simulink model "ARDroneWPTrackingSimulationRedBull"  (R2018b)
settings: Solver=ode1  StartTime=0.0  StopTime=150  FixedStep=t_samp  RelTol=1e-3  EnableMultiTasking=on
undefined symbols (not defined in the file): Gxd_A_obs, Gxd_B_obs, Gxd_C_obs, Gyawd_A_obs, Gyawd_B_obs, Gyawd_C_obs, Gyd_A_obs, Gyd_B_obs, Gyd_C_obs, Gzd_A_obs, Gzd_B_obs, Gzd_C_obs, K0_X, K0_Y, K0_yaw, K0_Z, K_X, K_Y, K_yaw, K_Z, KGe_X, KGe_Y, KGe_yaw, KGe_Z, ssH, ssPitch, ssPitch2U, ssRoll, ssRoll2V, ssYaw, t_samp, waypoint
libraries: simulink x3
CloseFcn:
  | rtwprivate ssgencode ModelCloseRequest Good_NL_model
settings Model: ExtModeTrigDuration=100000  Creator=Paul  LastModifiedBy=Henrique
settings DataIOCC: LimitDataPoints=on  SaveFormat=Array  TimeSaveName=time
settings OptimizationCC: ExpressionDepthLimit=2147483647  InitFltsAndDblsToZero=on
settings DebuggingCC: UnderspecifiedInitializationDetection=Classic  MergeDetectMultiDrivingBlocksExec=none  SolverPrmCheckMsg=warning  FcnCallInpInsideContextMsg=warning  StateNameClashWarn=warning  SFUnexpectedBacktrackingDiag=warning  SFNoUnconditionalDefaultTransitionDiag=warning  SFExecutionAtInitializationDiag=none
settings ModelReferenceCC: PropagateSignalLabelsOutOfModel=off
settings SFSimCC: SimUseLocalCustomCode=off
settings RTWCC: SystemTargetFile=sldrt.tlc  TemplateMakefile=sldrt.tmf  Description=Simulink Desktop Real-Time  RTWUseLocalCustomCode=off  RTWCompilerOptimization=on
settings CodeAppCC: MaxIdLength=95  StateflowObjectComments=on
settings SimulinkDesktopRealTimeCC: TargetPreCompLibLocation=D:\Programas\MATLAB 2018b\toolbox\sldrt\lib\win64  TargetLangStandard=C89/C90 (ANSI)  SupportVariableSizeSignals=off  PreserveStateflowLocalDataDimensions=off
settings ConfigComp: CovMetricSettings=dw  CovHtmlReporting=on  CovSaveCumulativeToWorkspaceVar=on  CovSaveSingleToWorkspaceVar=on  CovExternalEMLEnable=off

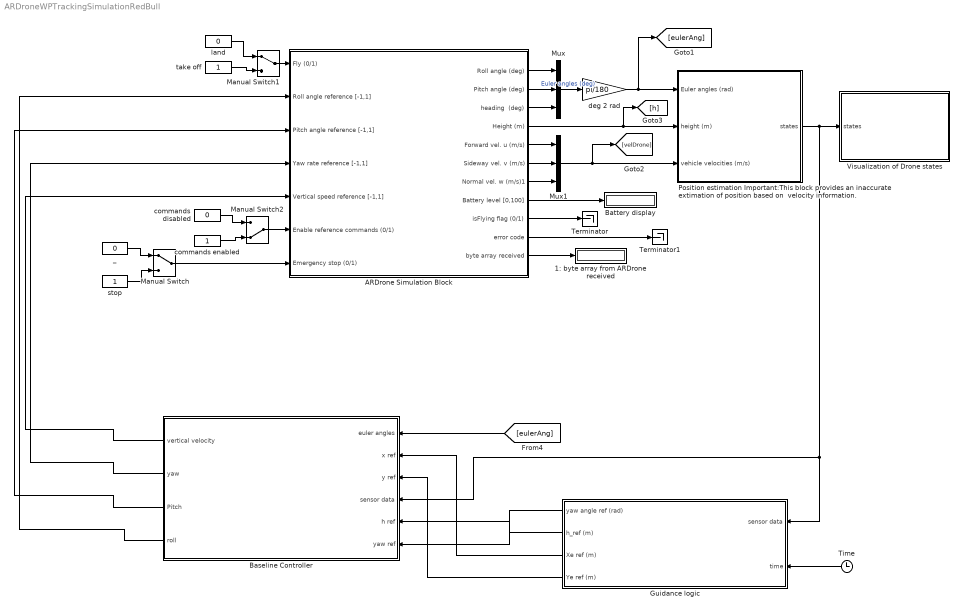
== system ARDroneWPTrackingSimulationRedBull ==
  "1: byte array from ARDrone received " : Display
  ARDrone Simulation Block : Subsystem  AncestorBlock=ARBlocks/ARDrone Simulation Block
  Baseline Controller : Subsystem  AncestorBlock=ARBlocks/Baseline Controller
  Battery display : Display
  Guidance logic : Subsystem  AncestorBlock=ARBlocks/Guidance logic
  Manual Switch : ManualSwitch
  Manual Switch1 : ManualSwitch
  Manual Switch2 : ManualSwitch  CurrentSetting=0
  Mux : Mux  Inputs=3
  Mux1 : Mux  Inputs=3
  "Position estimation Important:This block provides an inaccurate extimation of position based on  velocity information. " : Subsystem  AncestorBlock=|
      | ARBlocks/Position estimation
      | Important:This block provides an 
      | inaccurate extimation of position 
      | based on  velocity information.
  Terminator : Terminator
  Terminator1 : Terminator
  Time : Clock
  Visualization of Drone states : Subsystem
  _ : Constant  Value=0
  commands disabled : Constant  Value=0
  commands enabled : Constant
  deg 2 rad : Gain  Gain=pi/180
  land : Constant  Value=0
  stop : Constant
  take off : Constant
  wires:
  _/1 -> Manual Switch/1
  stop/1 -> Manual Switch/2
  land/1 -> Manual Switch1/1
  take off/1 -> Manual Switch1/2
  commands disabled/1 -> Manual Switch2/1
  commands enabled/1 -> Manual Switch2/2
  Manual Switch1/1 -> ARDrone Simulation Block/1(Fly (0/1))
  Manual Switch2/1 -> ARDrone Simulation Block/6(Enable reference commands (0/1))
  Manual Switch/1 -> ARDrone Simulation Block/7(Emergency stop (0/1))
  ARDrone Simulation Block/1(Roll angle (deg)) -> Mux/1
  ARDrone Simulation Block/2(Pitch angle (deg)) -> Mux/2
  ARDrone Simulation Block/5(Forward vel. u (m/s)) -> Mux1/1
  ARDrone Simulation Block/6(Sideway vel. v (m/s)) -> Mux1/2
  ARDrone Simulation Block/7(Normal vel. w (m/s)1) -> Mux1/3
  Mux/1 -> deg 2 rad/1  "Euler angles (deg)"
  ARDrone Simulation Block/8(Battery level [0,100]) -> Battery display/1
  deg 2 rad/1 -> "Position estimation Important:This block provides an inaccurate extimation of position based on  velocity information. "/1(Euler angles (rad)), [eulerAng]
  ARDrone Simulation Block/4(Height (m)) -> [h], "Position estimation Important:This block provides an inaccurate extimation of position based on  velocity information. "/2(height (m))
  ARDrone Simulation Block/3(heading  (deg)) -> Mux/3
  ARDrone Simulation Block/9(isFlying flag (0/1)) -> Terminator/1
  ARDrone Simulation Block/10(error code) -> Terminator1/1
  ARDrone Simulation Block/11(byte array received) -> "1: byte array from ARDrone received "/1
  "Position estimation Important:This block provides an inaccurate extimation of position based on  velocity information. "/1(states) -> Baseline Controller/4(sensor data), Guidance logic/1(sensor data), Visualization of Drone states/1(states)
  Mux1/1 -> [velDrone], "Position estimation Important:This block provides an inaccurate extimation of position based on  velocity information. "/3(vehicle velocities (m/s))
  [eulerAng] -> Baseline Controller/1(euler angles)
  Time/1 -> Guidance logic/2(time)
  Guidance logic/3(Xe ref (m)) -> Baseline Controller/2(x ref)
  Guidance logic/4(Ye ref (m)) -> Baseline Controller/3(y ref)
  Baseline Controller/1("vertical velocity ") -> ARDrone Simulation Block/5(Vertical speed reference [-1,1])
  Baseline Controller/2("yaw ") -> ARDrone Simulation Block/4(Yaw rate reference [-1,1])
  Baseline Controller/3("Pitch ") -> ARDrone Simulation Block/3(Pitch angle reference [-1,1])
  Baseline Controller/4("roll ") -> ARDrone Simulation Block/2(Roll angle reference [-1,1])
  Guidance logic/2(h_ref (m)) -> Baseline Controller/5(h ref)
  Guidance logic/1(yaw angle ref (rad)) -> Baseline Controller/6(yaw ref)

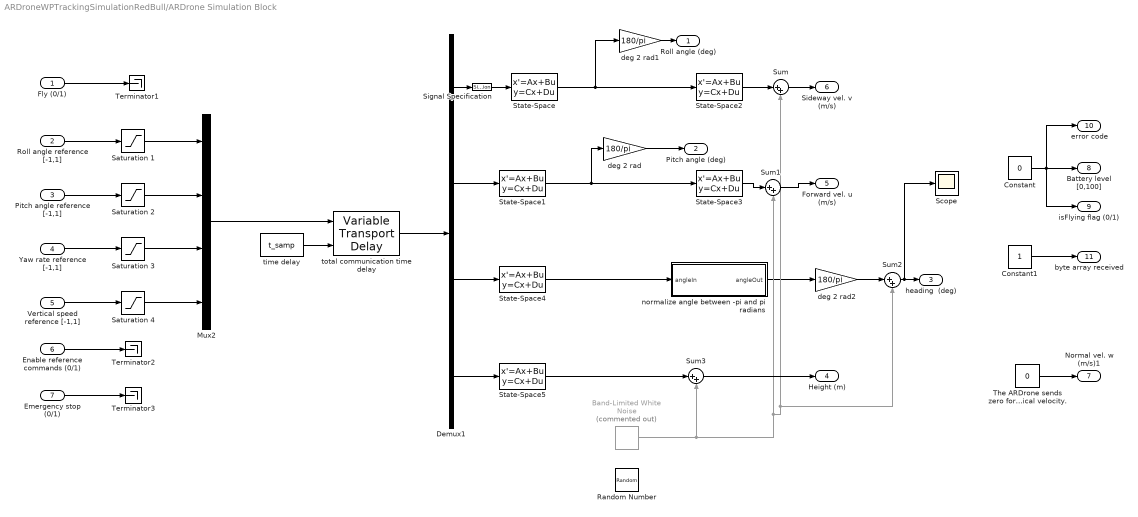
== system ARDroneWPTrackingSimulationRedBull/ARDrone Simulation Block ==
  Fly (0/1) : Inport
  Roll angle reference [-1,1] : Inport  Port=2
  Pitch angle reference [-1,1] : Inport  Port=3
  Yaw rate reference [-1,1] : Inport  Port=4
  Vertical speed reference [-1,1] : Inport  Port=5
  Enable reference commands (0/1) : Inport  Port=6
  Emergency stop (0/1) : Inport  Port=7
  Band-Limited White Noise : simulink/Sources/Band-Limited White Noise  Commented=on  Cov=[0.1]  Ts=0.065  seed=[23341]
  Constant : Constant  Value=0
  Constant1 : Constant
  Demux1 : Demux
  Mux2 : Mux
  Random Number : RandomNumber  SampleTime=0.065
  Saturation {1..4} (4 alike) : Saturate  UpperLimit=1  LowerLimit=-1
  Scope : Scope
  Signal Specification : SignalSpecification  Dimensions=1
  State-Space : StateSpace  A=ssRoll.a  B=ssRoll.b  C=ssRoll.c  D=ssRoll.d  InitialCondition=0
  State-Space1 : StateSpace  A=ssPitch.a  B=ssPitch.b  C=ssPitch.c  D=ssPitch.d  InitialCondition=0
  State-Space2 : StateSpace  A=ssRoll2V.a  B=ssRoll2V.b  C=ssRoll2V.c  D=ssRoll2V.d  InitialCondition=0
  State-Space3 : StateSpace  A=ssPitch2U.a  B=ssPitch2U.b  C=ssPitch2U.c  D=ssPitch2U.d  InitialCondition=0
  State-Space4 : StateSpace  A=ssYaw.a  B=ssYaw.b  C=ssYaw.c  D=ssYaw.d  InitialCondition=0
  State-Space5 : StateSpace  A=ssH.a  B=ssH.b  C=ssH.c  D=ssH.d  InitialCondition=0
  Sum{,1..3} (4 alike) : Sum  Inputs=|++
  Terminator1 : Terminator
  Terminator2 : Terminator
  Terminator3 : Terminator
  "The ARDrone sends zero for the vertical velocity. " : Constant  Value=0
  deg 2 rad : Gain  Gain=180/pi
  deg 2 rad1 : Gain  Gain=180/pi
  deg 2 rad2 : Gain  Gain=180/pi
  normalize angle between -pi and pi radians : MATLAB Function  TreatAsAtomicUnit=on
  time delay : Constant  Value=t_samp
  total communication time delay : VariableTransportDelay  MaximumDelay=10  InitialOutput=[0 0 0 0]  MaximumPoints=4096
  Roll angle (deg) : Outport
  Pitch angle (deg) : Outport  Port=2
  heading  (deg) : Outport  Port=3
  Height (m) : Outport  Port=4
  Forward vel. u (m/s) : Outport  Port=5
  Sideway vel. v (m/s) : Outport  Port=6
  Normal vel. w (m/s)1 : Outport  Port=7
  Battery level [0,100] : Outport  Port=8
  isFlying flag (0/1) : Outport  Port=9
  error code : Outport  Port=10
  byte array received : Outport  Port=11
  wires:
  "The ARDrone sends zero for the vertical velocity. "/1 -> Normal vel. w (m/s)1/1
  Constant1/1 -> byte array received/1
  deg 2 rad1/1 -> Roll angle (deg)/1
  deg 2 rad/1 -> Pitch angle (deg)/1
  Constant/1 -> Battery level [0,100]/1, error code/1, isFlying flag (0/1)/1
  normalize angle between -pi and pi radians/1(angleOut) -> deg 2 rad2/1
  Emergency stop (0/1)/1 -> Terminator3/1
  Enable reference commands (0/1)/1 -> Terminator2/1
  Fly (0/1)/1 -> Terminator1/1
  State-Space4/1 -> normalize angle between -pi and pi radians/1(angleIn)
  Demux1/3 -> State-Space4/1
  Demux1/2 -> State-Space1/1
  Saturation 4/1 -> Mux2/4
  Saturation 3/1 -> Mux2/3
  Saturation 2/1 -> Mux2/2
  Saturation 1/1 -> Mux2/1
  total communication time delay/1 -> Demux1/1
  Mux2/1 -> total communication time delay/1
  time delay/1 -> total communication time delay/2
  State-Space1/1 -> State-Space3/1, deg 2 rad/1
  State-Space/1 -> State-Space2/1, deg 2 rad1/1
  Demux1/4 -> State-Space5/1
  Vertical speed reference [-1,1]/1 -> Saturation 4/1
  Yaw rate reference [-1,1]/1 -> Saturation 3/1
  Pitch angle reference [-1,1]/1 -> Saturation 2/1
  Roll angle reference [-1,1]/1 -> Saturation 1/1
  Demux1/1 -> Signal Specification/1
  Signal Specification/1 -> State-Space/1
  State-Space2/1 -> Sum/1
  Sum/1 -> Sideway vel. v (m/s)/1
  Band-Limited White Noise/1 -> Sum3/2, Sum1/2, Sum2/2, Sum/2
  State-Space3/1 -> Sum1/1
  Sum1/1 -> Forward vel. u (m/s)/1
  Sum2/1 -> Scope/1, heading  (deg)/1
  deg 2 rad2/1 -> Sum2/1
  State-Space5/1 -> Sum3/1
  Sum3/1 -> Height (m)/1

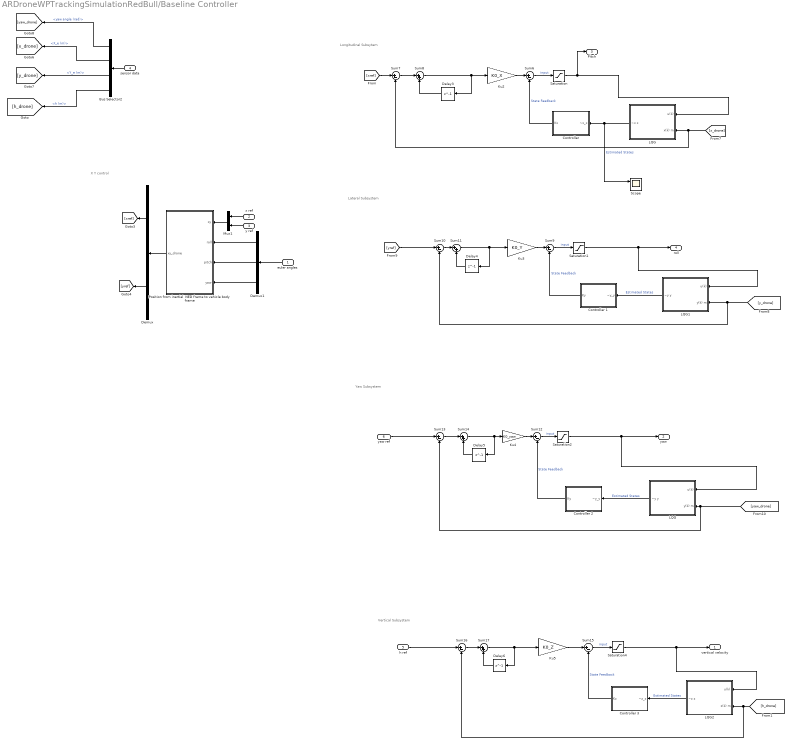
== system ARDroneWPTrackingSimulationRedBull/Baseline Controller ==
  note: Vertical Subsystem
  note: Yaw Subsystem
  note: Lateral Subsystem
  note: Longitudinal Subsytem
  note: X Y control
  euler angles : Inport
  x ref : Inport  Port=2
  y ref : Inport  Port=3
  sensor data : Inport  Port=4
  h ref : Inport  Port=5
  yaw ref : Inport  Port=6
  Bus Selector2 : BusSelector  OutputSignals=yaw angle (rad),X_e (m),Y_e (m),h (m)
  "Controller " : Subsystem
  Controller 1 : Subsystem
  Controller 2 : Subsystem
  Controller 3 : Subsystem
  Delay{3..6} (4 alike) : Delay  DelayLength=1  InitialCondition=0
  Demux : Demux  Outputs=2
  Demux1 : Demux  Outputs=3
  Ku2 : Gain  Gain=K0_X
  Ku3 : Gain  Gain=K0_Y
  Ku4 : Gain  Gain=K0_yaw
  Ku5 : Gain  Gain=K0_Z
  LQG : Subsystem
  "LQG " : Subsystem
  LQG1 : Subsystem
  LQG2 : Subsystem
  Mux1 : Mux  Inputs=2
  Position from inertial  NED frame to vehicle body frame : MATLAB Function  TreatAsAtomicUnit=on
  Saturation : Saturate  UpperLimit=2  LowerLimit=-1.2
  Saturation1 : Saturate  UpperLimit=1.2  LowerLimit=-1.2
  Saturation2 : Saturate  UpperLimit=1.2  LowerLimit=-1.2
  Saturation4 : Saturate  UpperLimit=1.2  LowerLimit=-1.2
  Scope : Scope  NumInputPorts=2
  Sum{6..7,9..10,12..13,15..16} (8 alike) : Sum  Inputs=|+-
  Sum{8,11,14,17} (4 alike) : Sum  Inputs=|++
  "vertical velocity " : Outport
  "yaw " : Outport  Port=2
  "Pitch " : Outport  Port=3
  "roll " : Outport  Port=4
  wires:
  Mux1/1 -> Position from inertial  NED frame to vehicle body frame/1(xy)
  x ref/1 -> Mux1/1
  y ref/1 -> Mux1/2
  Position from inertial  NED frame to vehicle body frame/1(xy_drone) -> Demux/1
  Demux1/1 -> Position from inertial  NED frame to vehicle body frame/2(roll)
  Demux1/2 -> Position from inertial  NED frame to vehicle body frame/3(pitch)
  Demux1/3 -> Position from inertial  NED frame to vehicle body frame/4(yaw)
  euler angles/1 -> Demux1/1
  Bus Selector2/1 -> [yaw_drone]  "<yaw angle (rad)>"
  Bus Selector2/3 -> [y_drone]  "<Y_e (m)>"
  sensor data/1 -> Bus Selector2/1
  Bus Selector2/4 -> [h_drone]  "<h (m)>"
  Bus Selector2/2 -> [x_drone]  "<X_e (m)>"
  Delay3/1 -> Sum8/2
  Ku2/1 -> Sum6/1
  LQG/1("~x x ") -> Scope/1, "Controller "/1(~x_x)  "Estimated States"
  "Controller "/1(Kx) -> Sum6/2  "State Feedback"
  Sum8/1 -> Ku2/1, Delay3/1
  [xref] -> Sum7/1
  Saturation/1 -> "Pitch "/1, LQG/1(u(k))
  [x_drone] -> Sum7/2, LQG/2(x(k) m)
  Sum7/1 -> Sum8/1
  Sum6/1 -> Saturation/1  "input"
  Demux/1 -> [xref]
  Ku3/1 -> Sum9/1
  Controller 1/1(Ky) -> Sum9/2  "State Feedback"
  Sum11/1 -> Delay4/1, Ku3/1
  [yref] -> Sum10/1
  Sum10/1 -> Sum11/1
  Delay4/1 -> Sum11/2
  LQG1/1("~y y ") -> Controller 1/1(~y_y)  "Estimated States"
  [y_drone] -> Sum10/2, LQG1/2(y(k) m)
  Saturation1/1 -> "roll "/1, LQG1/1(u(k))
  Sum9/1 -> Saturation1/1  "input"
  Delay5/1 -> Sum14/2
  Saturation2/1 -> "yaw "/1, "LQG "/1(u(k))
  Sum14/1 -> Delay5/1, Ku4/1
  "LQG "/1("~y y ") -> Controller 2/1(~y_y)  "Estimated States"
  Sum12/1 -> Saturation2/1  "input"
  [yaw_drone] -> Sum13/2, "LQG "/2(y(k) m)
  Ku4/1 -> Sum12/1
  Sum13/1 -> Sum14/1
  Controller 2/1(Ky) -> Sum12/2  "State Feedback"
  yaw ref/1 -> Sum13/1
  Sum17/1 -> Ku5/1, Delay6/1
  Sum16/1 -> Sum17/1
  Controller 3/1(Kz) -> Sum15/2  "State Feedback"
  Sum15/1 -> Saturation4/1  "input"
  Saturation4/1 -> "vertical velocity "/1, LQG2/1(u(k))
  LQG2/1("~z z ") -> Controller 3/1(~z_z)  "Estimated States"
  Ku5/1 -> Sum15/1
  h ref/1 -> Sum16/1
  Delay6/1 -> Sum17/2
  [h_drone] -> Sum16/2, LQG2/2(z(k) m)
  Demux/2 -> [yref]

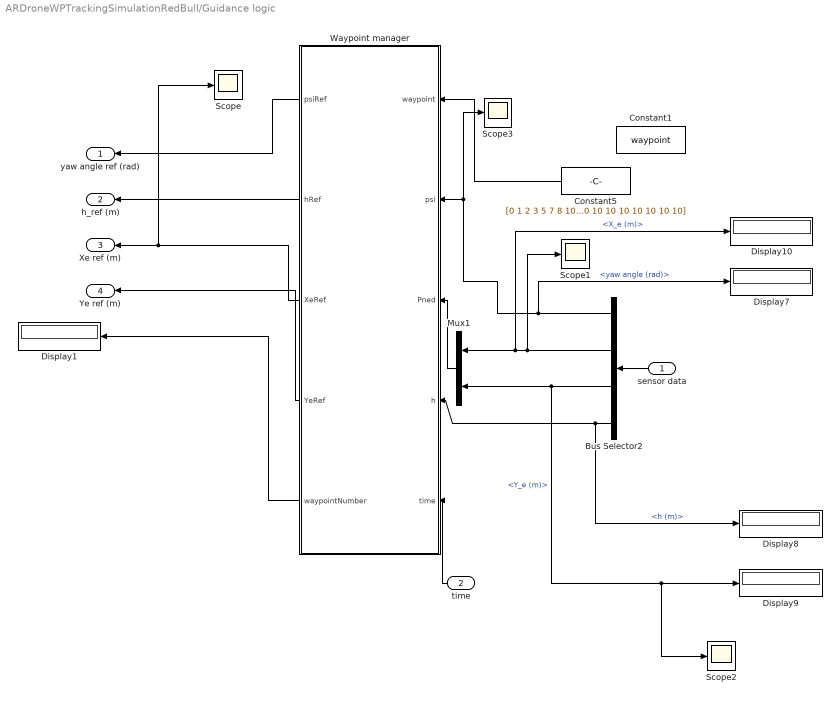
== system ARDroneWPTrackingSimulationRedBull/Guidance logic ==
  sensor data : Inport
  time : Inport  Port=2
  Bus Selector2 : BusSelector  OutputSignals=yaw angle (rad),X_e (m),Y_e (m),h (m)
  Constant1 : Constant  Value=waypoint  VectorParams1D=off
  Constant5 : Constant  Value="[0 1 2 3 5 7 8 10 11 12 13; 0 2 2 5 5 -1 -1 -2 -2 1 1; 1 2 5 2 2 1 2 3 1 1 1; 0 -0.1 0 0 0 0 0 0 0 0 0;  10 10 10 10 10 10 10 10 10 10 10]"  VectorParams1D=off
  Display{1,7..10} (5 alike) : Display
  Mux1 : Mux  Inputs=2
  Scope{,1..3} (4 alike) : Scope
  "Waypoint manager " : MATLAB Function  TreatAsAtomicUnit=on
  yaw angle ref (rad) : Outport
  h_ref (m) : Outport  Port=2
  Xe ref (m) : Outport  Port=3
  Ye ref (m) : Outport  Port=4
  wires:
  "Waypoint manager "/3(XeRef) -> Scope/1, Xe ref (m)/1
  "Waypoint manager "/5(waypointNumber) -> Display1/1
  Bus Selector2/1 -> Display7/1, Scope3/1, "Waypoint manager "/2(psi)  "<yaw angle (rad)>"
  "Waypoint manager "/1(psiRef) -> yaw angle ref (rad)/1
  Bus Selector2/2 -> Scope1/1, Mux1/1, Display10/1  "<X_e (m)>"
  Mux1/1 -> "Waypoint manager "/3(Pned)
  "Waypoint manager "/4(YeRef) -> Ye ref (m)/1
  Bus Selector2/3 -> Scope2/1, Display9/1, Mux1/2  "<Y_e (m)>"
  time/1 -> "Waypoint manager "/5(time)
  Bus Selector2/4 -> Display8/1, "Waypoint manager "/4(h)  "<h (m)>"
  Constant5/1 -> "Waypoint manager "/1(waypoint)
  "Waypoint manager "/2(hRef) -> h_ref (m)/1
  sensor data/1 -> Bus Selector2/1

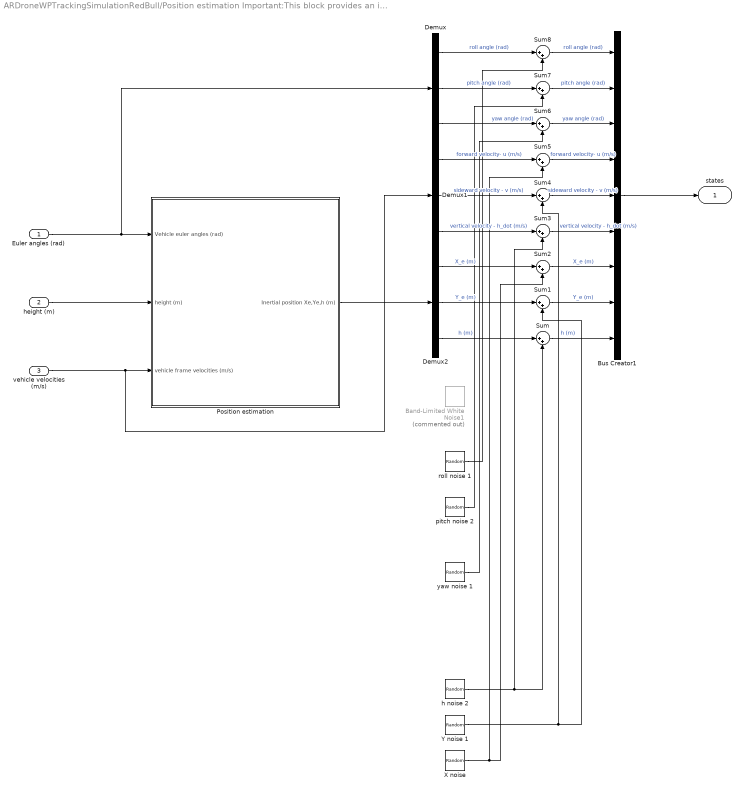
== system ARDroneWPTrackingSimulationRedBull/Position estimation Important:This block provides an inaccurate extimation of position based on  velocity information.  ==
  Euler angles (rad) : Inport
  height (m) : Inport  Port=2
  vehicle velocities (m/s) : Inport  Port=3
  Band-Limited White Noise1 : simulink/Sources/Band-Limited White Noise  Commented=on  Cov=.000001  Ts=0.065  seed=[124123]
  Bus Creator1 : BusCreator  Inputs=9
  Demux : Demux  Outputs=3
  Demux1 : Demux  Outputs=3
  Demux2 : Demux  Outputs=3
  Position estimation : Subsystem
  Sum{,1..8} (9 alike) : Sum  Inputs=|++
  "X noise " : RandomNumber  Variance=0.001166  SampleTime=t_samp
  Y noise 1 : RandomNumber  Variance=0.000961  SampleTime=t_samp
  h noise 2 : RandomNumber  Variance=0.002762  SampleTime=t_samp
  pitch noise 2 : RandomNumber  Variance=0.000238  SampleTime=t_samp
  roll noise 1 : RandomNumber  Variance=0.000444  SampleTime=t_samp
  yaw noise 1 : RandomNumber  Variance=0.000061  SampleTime=t_samp
  states : Outport
  wires:
  height (m)/1 -> Position estimation/2(height (m))
  Bus Creator1/1 -> states/1
  Position estimation/1(Inertial position Xe,Ye,h (m)) -> Demux2/1
  Euler angles (rad)/1 -> Demux/1, Position estimation/1(Vehicle euler angles (rad))
  vehicle velocities (m/s)/1 -> Position estimation/3(vehicle frame velocities (m/s)), Demux1/1
  Demux2/3 -> Sum/1  "h (m)"
  Sum/1 -> Bus Creator1/9  "h (m)"
  Demux2/2 -> Sum1/1  "Y_e (m)"
  Sum1/1 -> Bus Creator1/8  "Y_e (m)"
  Demux2/1 -> Sum2/1  "X_e (m)"
  Demux1/3 -> Sum3/1  "vertical velocity - h_dot (m/s)"
  Demux1/2 -> Sum4/1  "sideward velocity - v (m/s)"
  Demux1/1 -> Sum5/1  "forward velocity- u (m/s)"
  Demux/3 -> Sum6/1  "yaw angle (rad)"
  Demux/1 -> Sum8/1  "roll angle (rad)"
  Demux/2 -> Sum7/1  "pitch angle (rad)"
  Sum8/1 -> Bus Creator1/1  "roll angle (rad)"
  Sum7/1 -> Bus Creator1/2  "pitch angle (rad)"
  Sum6/1 -> Bus Creator1/3  "yaw angle (rad)"
  Sum5/1 -> Bus Creator1/4  "forward velocity- u (m/s)"
  Sum4/1 -> Bus Creator1/5  "sideward velocity - v (m/s)"
  Sum3/1 -> Bus Creator1/6  "vertical velocity - h_dot (m/s)"
  Sum2/1 -> Bus Creator1/7  "X_e (m)"
  "X noise "/1 -> Sum5/2, Sum2/2
  Y noise 1/1 -> Sum4/2, Sum1/2
  h noise 2/1 -> Sum3/2, Sum/2
  roll noise 1/1 -> Sum8/2
  pitch noise 2/1 -> Sum7/2
  yaw noise 1/1 -> Sum6/2

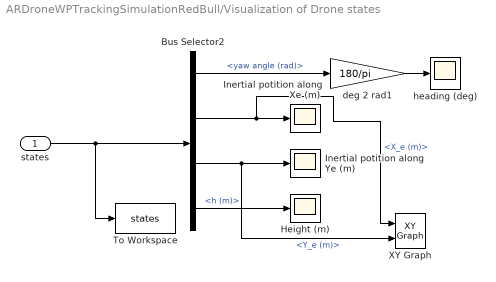
== system ARDroneWPTrackingSimulationRedBull/Visualization of Drone states ==
  states : Inport
  Bus Selector2 : BusSelector  OutputSignals=yaw angle (rad),X_e (m),Y_e (m),h (m)
  Height (m) : Scope
  Inertial potition along Xe (m) : Scope
  Inertial potition along Ye (m) : Scope
  To Workspace : ToWorkspace  VariableName=states  SaveFormat=Structure With Time  SampleTime=-1
  XY Graph : simulink/Sinks/XY Graph  xmin=-3  xmax=20  ymin=-10  ymax=10  st=t_samp
  deg 2 rad1 : Gain  Gain=180/pi
  heading (deg) : Scope
  wires:
  states/1 -> To Workspace/1, Bus Selector2/1
  Bus Selector2/1 -> deg 2 rad1/1  "<yaw angle (rad)>"
  Bus Selector2/2 -> XY Graph/1, Inertial potition along Xe (m)/1  "<X_e (m)>"
  Bus Selector2/3 -> XY Graph/2, Inertial potition along Ye (m)/1  "<Y_e (m)>"
  Bus Selector2/4 -> Height (m)/1  "<h (m)>"
  deg 2 rad1/1 -> heading (deg)/1

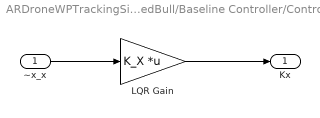
== system ARDroneWPTrackingSimulationRedBull/Baseline Controller/Controller  ==
  ~x_x : Inport
  "LQR Gain " : Gain  Gain=K_X  Multiplication=Matrix(K*u) (u vector)
  Kx : Outport
  wires:
  ~x_x/1 -> "LQR Gain "/1
  "LQR Gain "/1 -> Kx/1

== system ARDroneWPTrackingSimulationRedBull/Baseline Controller/Controller 1 ==
  ~y_y : Inport
  Gain : Gain  Gain=K_Y  Multiplication=Matrix(K*u) (u vector)
  Ky : Outport
  wires:
  ~y_y/1 -> Gain/1
  Gain/1 -> Ky/1

== system ARDroneWPTrackingSimulationRedBull/Baseline Controller/Controller 2 ==
  ~y_y : Inport
  Gain : Gain  Gain=K_yaw  Multiplication=Matrix(K*u) (u vector)
  Ky : Outport
  wires:
  ~y_y/1 -> Gain/1
  Gain/1 -> Ky/1

== system ARDroneWPTrackingSimulationRedBull/Baseline Controller/Controller 3 ==
  ~z_z : Inport
  Gain : Gain  Gain=K_Z  Multiplication=Matrix(K*u) (u vector)
  Kz : Outport
  wires:
  ~z_z/1 -> Gain/1
  Gain/1 -> Kz/1

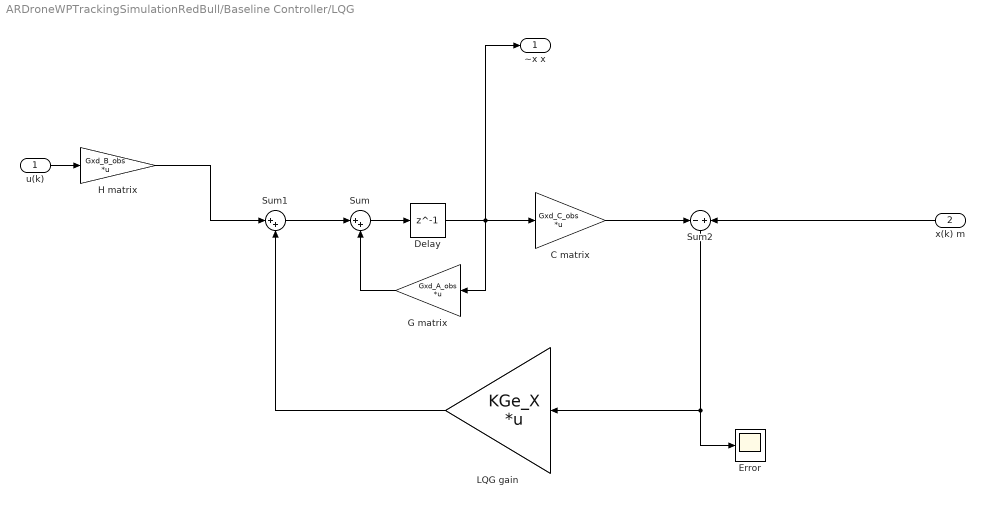
== system ARDroneWPTrackingSimulationRedBull/Baseline Controller/LQG ==
  u(k) : Inport
  x(k) m : Inport  Port=2
  C matrix : Gain  Gain=Gxd_C_obs  Multiplication=Matrix(K*u)
  Delay : Delay  DelayLength=1  InitialCondition=0  SampleTime=t_samp
  Error : Scope
  G matrix : Gain  Gain=Gxd_A_obs  Multiplication=Matrix(K*u)
  H matrix : Gain  Gain=Gxd_B_obs  Multiplication=Matrix(K*u)
  LQG gain : Gain  Gain=KGe_X  Multiplication=Matrix(K*u)
  Sum : Sum  Inputs=|++
  Sum1 : Sum  Inputs=|++
  Sum2 : Sum  Inputs=-+
  "~x x " : Outport
  wires:
  C matrix/1 -> Sum2/1
  x(k) m/1 -> Sum2/2
  H matrix/1 -> Sum1/1
  Sum/1 -> Delay/1
  u(k)/1 -> H matrix/1
  G matrix/1 -> Sum/2
  Sum2/1 -> Error/1, LQG gain/1
  LQG gain/1 -> Sum1/2
  Delay/1 -> "~x x "/1, G matrix/1, C matrix/1
  Sum1/1 -> Sum/1

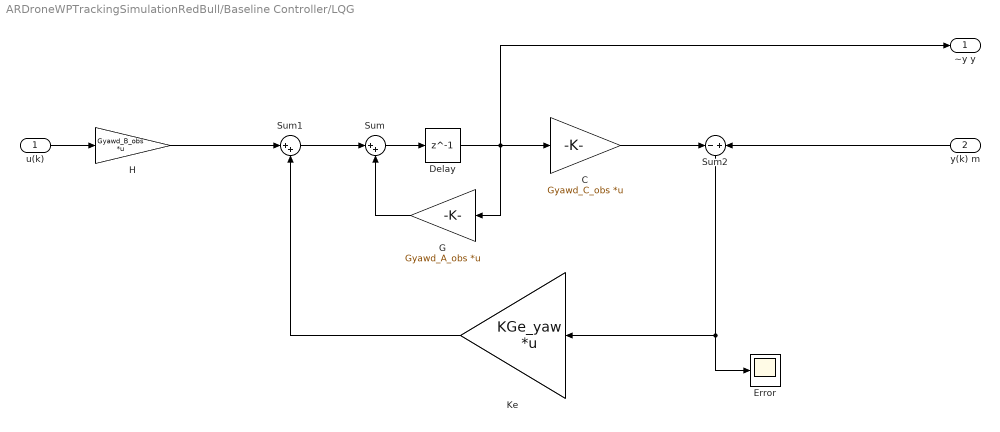
== system ARDroneWPTrackingSimulationRedBull/Baseline Controller/LQG  ==
  u(k) : Inport
  y(k) m : Inport  Port=2
  C : Gain  Gain=Gyawd_C_obs  Multiplication=Matrix(K*u)
  Delay : Delay  DelayLength=1  InitialCondition=0  SampleTime=t_samp
  Error : Scope
  G : Gain  Gain=Gyawd_A_obs  Multiplication=Matrix(K*u)
  H : Gain  Gain=Gyawd_B_obs  Multiplication=Matrix(K*u)
  Ke : Gain  Gain=KGe_yaw  Multiplication=Matrix(K*u)
  Sum : Sum  Inputs=|++
  Sum1 : Sum  Inputs=|++
  Sum2 : Sum  Inputs=-+
  "~y y " : Outport
  wires:
  C/1 -> Sum2/1
  y(k) m/1 -> Sum2/2
  H/1 -> Sum1/1
  Sum/1 -> Delay/1
  u(k)/1 -> H/1
  G/1 -> Sum/2
  Sum2/1 -> Error/1, Ke/1
  Sum1/1 -> Sum/1
  Ke/1 -> Sum1/2
  Delay/1 -> "~y y "/1, G/1, C/1

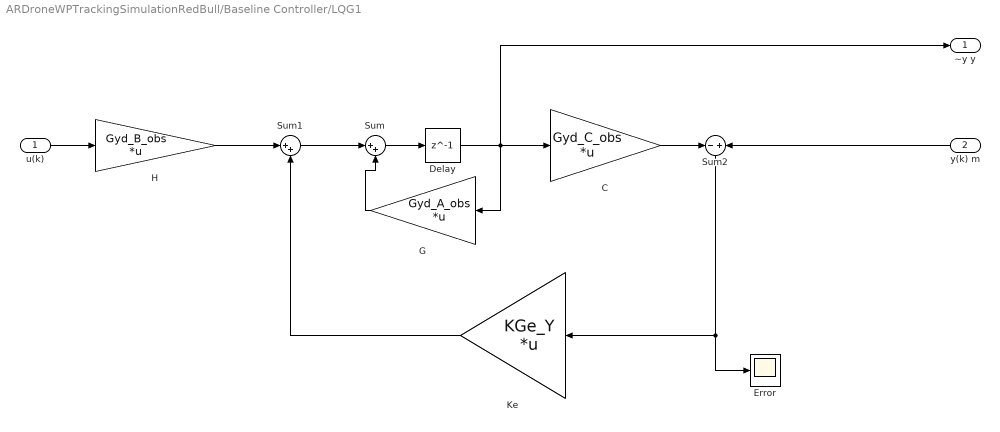
== system ARDroneWPTrackingSimulationRedBull/Baseline Controller/LQG1 ==
  u(k) : Inport
  y(k) m : Inport  Port=2
  C : Gain  Gain=Gyd_C_obs  Multiplication=Matrix(K*u)
  Delay : Delay  DelayLength=1  InitialCondition=0  SampleTime=t_samp
  Error : Scope
  G : Gain  Gain=Gyd_A_obs  Multiplication=Matrix(K*u)
  H : Gain  Gain=Gyd_B_obs  Multiplication=Matrix(K*u)
  Ke : Gain  Gain=KGe_Y  Multiplication=Matrix(K*u)
  Sum : Sum  Inputs=|++
  Sum1 : Sum  Inputs=|++
  Sum2 : Sum  Inputs=-+
  "~y y " : Outport
  wires:
  C/1 -> Sum2/1
  y(k) m/1 -> Sum2/2
  H/1 -> Sum1/1
  Sum/1 -> Delay/1
  u(k)/1 -> H/1
  G/1 -> Sum/2
  Sum2/1 -> Error/1, Ke/1
  Sum1/1 -> Sum/1
  Ke/1 -> Sum1/2
  Delay/1 -> "~y y "/1, C/1, G/1

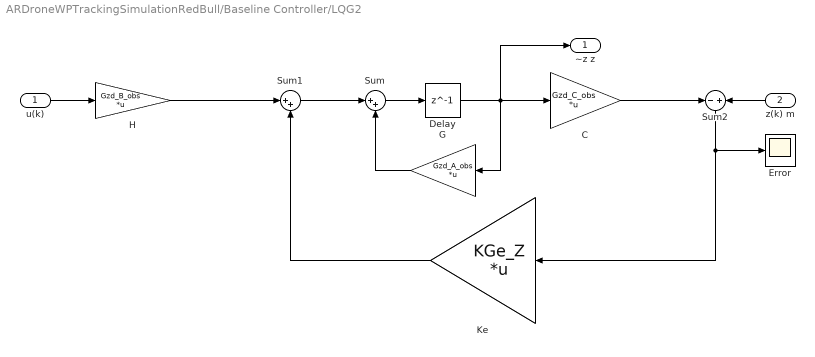
== system ARDroneWPTrackingSimulationRedBull/Baseline Controller/LQG2 ==
  u(k) : Inport
  z(k) m : Inport  Port=2
  C : Gain  Gain=Gzd_C_obs  Multiplication=Matrix(K*u)
  Delay : Delay  DelayLength=1  InitialCondition=0  SampleTime=t_samp
  Error : Scope
  G : Gain  Gain=Gzd_A_obs  Multiplication=Matrix(K*u)
  H : Gain  Gain=Gzd_B_obs  Multiplication=Matrix(K*u)
  Ke : Gain  Gain=KGe_Z  Multiplication=Matrix(K*u)
  Sum : Sum  Inputs=|++
  Sum1 : Sum  Inputs=|++
  Sum2 : Sum  Inputs=-+
  "~z z " : Outport
  wires:
  C/1 -> Sum2/1
  z(k) m/1 -> Sum2/2
  H/1 -> Sum1/1
  Sum/1 -> Delay/1
  u(k)/1 -> H/1
  G/1 -> Sum/2
  Sum2/1 -> Ke/1, Error/1
  Sum1/1 -> Sum/1
  Ke/1 -> Sum1/2
  Delay/1 -> G/1, "~z z "/1, C/1

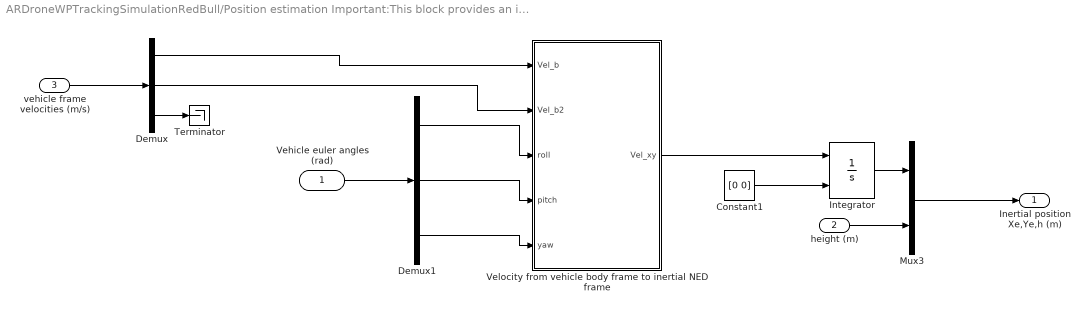
== system ARDroneWPTrackingSimulationRedBull/Position estimation Important:This block provides an inaccurate extimation of position based on  velocity information. /Position estimation ==
  Vehicle euler angles (rad) : Inport
  height (m) : Inport  Port=2
  vehicle frame velocities (m/s) : Inport  Port=3
  Constant1 : Constant  Value=[0 0]
  Demux : Demux  Outputs=3
  Demux1 : Demux  Outputs=3
  Integrator : Integrator  InitialConditionSource=external
  Mux3 : Mux  Inputs=2
  Terminator : Terminator
  Velocity from vehicle body frame to inertial NED  frame : MATLAB Function  TreatAsAtomicUnit=on
  Inertial position Xe,Ye,h (m) : Outport
  wires:
  Mux3/1 -> Inertial position Xe,Ye,h (m)/1
  height (m)/1 -> Mux3/2
  Vehicle euler angles (rad)/1 -> Demux1/1
  vehicle frame velocities (m/s)/1 -> Demux/1
  Integrator/1 -> Mux3/1
  Constant1/1 -> Integrator/2
  Velocity from vehicle body frame to inertial NED  frame/1(Vel_xy) -> Integrator/1
  Demux/1 -> Velocity from vehicle body frame to inertial NED  frame/1(Vel_b)
  Demux/2 -> Velocity from vehicle body frame to inertial NED  frame/2(Vel_b2)
  Demux/3 -> Terminator/1
  Demux1/1 -> Velocity from vehicle body frame to inertial NED  frame/3(roll)
  Demux1/2 -> Velocity from vehicle body frame to inertial NED  frame/4(pitch)
  Demux1/3 -> Velocity from vehicle body frame to inertial NED  frame/5(yaw)

== matlab function ARDroneWPTrackingSimulationRedBull/Baseline Controller/Position from inertial  NED frame to vehicle body frame ==
  data: xy input; roll input; pitch input; yaw input; xy_drone output
function xy_drone = fcn(xy , roll, pitch, yaw)
%#codegen
T = [cos(yaw)*cos(pitch) (sin(roll)*sin(pitch)*cos(yaw) - cos(roll)*sin(yaw)); 
    cos(pitch)*sin(yaw) (sin(roll)*sin(pitch)*sin(yaw) + cos(roll)*cos(yaw))] ; 

xy_drone = (T')*xy(1:2,1);

== matlab function ARDroneWPTrackingSimulationRedBull/ARDrone Simulation Block/normalize angle between -pi and pi radians ==
  data: angleIn input; angleOut output
function angleOut = fcn(angleIn)
%#codegen

angleOut = mod(angleIn, 2*pi) ;
if angleOut > pi
    angleOut = -2*pi + angleOut ; 
end

== matlab function ARDroneWPTrackingSimulationRedBull/Position estimation Important:This block provides an inaccurate extimation of position based on  velocity information. /Position estimation/Velocity from vehicle body frame to inertial NED  frame ==
  data: Vel_b input; Vel_b2 input; roll input; pitch input; yaw input; Vel_xy output
function Vel_xy = fcn(Vel_b, Vel_b2 , roll, pitch, yaw)
%#codegen
T = [cos(yaw)*cos(pitch) (sin(roll)*sin(pitch)*cos(yaw) - cos(roll)*sin(yaw)); 
    cos(pitch)*sin(yaw) (sin(roll)*sin(pitch)*sin(yaw) + cos(roll)*cos(yaw))] ; 
Vel_xy = T*[Vel_b; Vel_b2];

== matlab function ARDroneWPTrackingSimulationRedBull/Guidance logic/Waypoint manager  ==
  settings: updateMethod=DISCRETE
  data: psiRef output; hRef output; waypoint input; psi input; Pned input; h input; XeRef output; YeRef output; time input; waypointNumber output
function [psiRef, hRef,  XeRef, YeRef, waypointNumber]       = fcn(waypoint, psi, Pned, h, time )
%#codegen

% Waypoint matrix contains final position, orientatoin, and waiting time.

% Number of waypoints
nPoints = size(waypoint, 2) ;

% Persitent variable used to keep trak of next waypoint
persistent wpointer;

% Time zero for each waypoint. This is used to wait at a desired position.
persistent t0 ;

% Init. persistent variables
if isempty(wpointer)
    wpointer = 1;
end

if isempty(t0)
    t0 = 0;
end

% A waypoint is reached if the distance between the desired waypoint and 
% the vehicle is less than 0.3 m in the XY plane, less than 0.3 m in height, 
% and less than 5 degrees in  heading. 

if ( norm(Pned(1:2,1) - waypoint(1:2, wpointer) )< 0.3 && ...
        norm(h - waypoint(3, wpointer)) < 0.3  && norm(psi - waypoint(4, wpointer) )< 5*pi/180   )
    
    if(wpointer ~= nPoints)
        
        if (t0 ==0)
            t0 = time;
        else
            if (time - t0 > waypoint(5, wpointer))
                
                 if(wpointer < nPoints)
                    wpointer = wpointer+ 1;
                    t0 = 0;
                 end
                
            end
        end
        
             
    end
    
       
    
end


%% Outputs:
hRef = waypoint(3, wpointer) ;
psiRef = waypoint(4, wpointer) ;
XeRef = waypoint(1, wpointer) ;
YeRef = waypoint(2, wpointer) ;
waypointNumber = wpointer ;
